simulink model "miniprojectr12"  (R2015a)
settings: Solver=ode45  StartTime=0.0  StopTime=.1  RelTol=1e-3
undefined symbols (not defined in the file): D1, Delta
libraries: powerlib x16, dspstat3 x11, powerlib_meascontrol x4
settings Model: Creator=ASUS  LastModifiedBy=ASUS

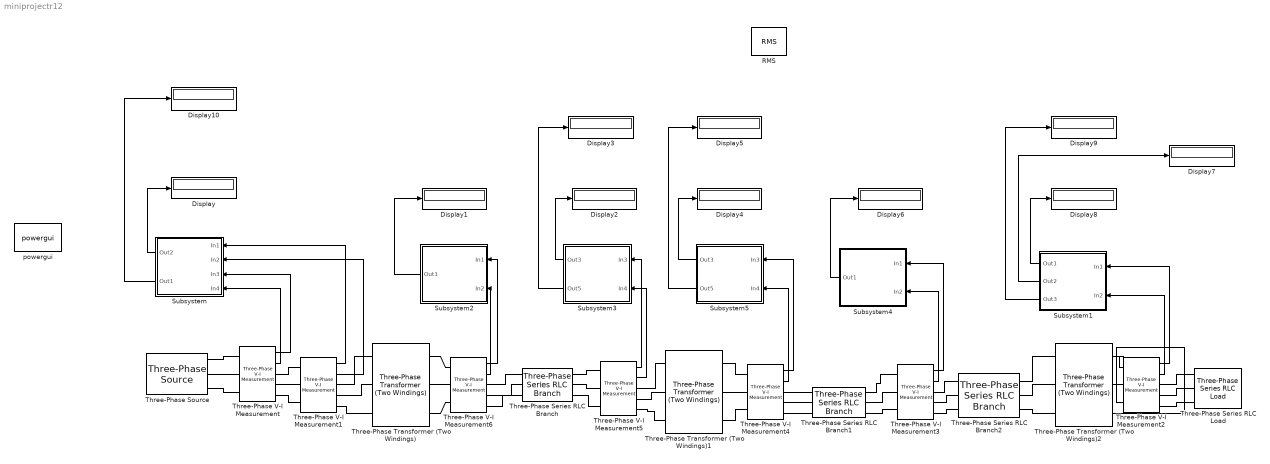
== system miniprojectr12 ==
  Display{,1..10} (11 alike) : Display
  RMS : powerlib_meascontrol/Measurements/RMS  TrueRMS=on  Freq=60  RMSInit=120  Ts=0
  Subsystem : Subsystem
  Subsystem1 : Subsystem
  Subsystem2 : Subsystem
  Subsystem3 : Subsystem
  Subsystem4 : Subsystem
  Subsystem5 : Subsystem
  Three-Phase Series RLC Branch : powerlib/Elements/Three-Phase Series RLC Branch  LConnTagsString=A|B|C  RConnTagsString=A|B|C  BranchType=RL  Resistance=271*0.01  Inductance=271*0.01  Capacitance=1e-6  Measurements=None
  Three-Phase Series RLC Branch1 : powerlib/Elements/Three-Phase Series RLC Branch  LConnTagsString=A|B|C  RConnTagsString=A|B|C  BranchType=RL  Resistance=271*0.01  Inductance=271*0.01  Capacitance=1e-6  Measurements=None
  Three-Phase Series RLC Branch2 : powerlib/Elements/Three-Phase Series RLC Branch  LConnTagsString=A|B|C  RConnTagsString=A|B|C  BranchType=RL  Resistance=271*0.01  Inductance=271*0.01  Capacitance=1e-6  Measurements=None
  Three-Phase Series RLC Load : powerlib/Elements/Three-Phase Series RLC Load  LConnTagsString=A|B|C  Configuration=Y (grounded)  NominalVoltage=1000  NominalFrequency=50  ActivePower=1e6  InductivePower=0.5e6  CapacitivePower=0  Measurements=None  LoadType=constant Z
  Three-Phase Transformer (Two Windings) : powerlib/Elements/Three-Phase Transformer (Two Windings)  Winding1Connection=Delta (D1)  Winding2Connection=Yg  CoreType=Three single-phase transformers  SetSaturation=off  Hysteresis=off  DataFile='hysteresis'  SetInitialFlux=off  Measurements=None  UNITS=pu  NominalPower=[ 250e6 , 50 ]  Winding1=[ 11e3 , 0.002 , 0.08 ]  Winding2=[ 230e3 , 0.002 , 0.08 ]  Rm=500  Lm=500  L0=0.5  Saturation=[ 0,0 ; 0.0024,1.2 ; 1.0,1.52 ]  InitialFluxes=[ 0.8 , -0.8 , 0.7 ]  MoreParameters=off  BreakLoop=off  DataType=off  TransfoNumber=1
  Three-Phase Transformer (Two Windings)1 : powerlib/Elements/Three-Phase Transformer (Two Windings)  Winding1Connection=Yg  Winding2Connection=Delta (D1)  CoreType=Three single-phase transformers  SetSaturation=off  Hysteresis=off  DataFile='hysteresis'  SetInitialFlux=off  Measurements=None  UNITS=SI  NominalPower=[ 450e6 , 50 ]  Winding1=[230e3 5.5555e-09 1.5636e-12]  Winding2=[11e3 2.7638e+09 7.7788e+05]  Rm=0.0013889  Lm=9.7726e-09  L0=2.2105e-06  Saturation=[0 0;4.3199e+08 4.2217;1.8e+11 5.3475]  InitialFluxes=[2.8144 -2.8144 2.4627]  MoreParameters=off  BreakLoop=off  DataType=on  TransfoNumber=1
  Three-Phase Transformer (Two Windings)2 : powerlib/Elements/Three-Phase Transformer (Two Windings)  Winding1Connection=Yg  Winding2Connection=Yg  CoreType=Three single-phase transformers  SetSaturation=off  Hysteresis=off  DataFile='hysteresis'  SetInitialFlux=off  Measurements=None  UNITS=pu  NominalPower=[ 450e6 , 50 ]  Winding1=[ 11000 , 0.002 , 0.08 ]  Winding2=[ 400 , 0.002 , 0.08 ]  Rm=500  Lm=500  L0=0.5  Saturation=[ 0,0 ; 0.0024,1.2 ; 1.0,1.52 ]  InitialFluxes=[ 0.8 , -0.8 , 0.7 ]  MoreParameters=off  BreakLoop=off  DataType=off  TransfoNumber=1
  Three-Phase V-I Measurement{,1..6} (7 alike) : powerlib/Measurements/Three-Phase V-I Measurement  VoltageMeasurement=phase-to-ground  SetLabelV=off  LabelV=Vabc  Vpu=off  VpuLL=off  CurrentMeasurement=yes  SetLabelI=off  LabelI=Iabc  Ipu=off  Pbase=100e6  Vbase=500e3  OutputType=Complex  PhasorSimulation=off  PSBequivalent=0
  Three-Phase Source : powerlib/Electrical Sources/Three-Phase Source  Voltage=11000  PhaseAngle=0  Frequency=50  InternalConnection=Yg  SpecifyImpedance=off  Resistance=0  Inductance=0  ShortCircuitLevel=100e6  BaseVoltage=25e3  XRratio=7  BusType=swing  Pref=0  Qref=0  Qmin=-inf  Qmax=inf
  powergui : powerlib/powergui  Priority=1  SimulationMode=Continuous  SolverType=Tustin/Backward Euler (TBE)  SampleTime=50e-6  frequency=60  SPID=off  DisableSnubberDevices=off  DisableRonSwitches=off  DisableVfSwitches=off  SwTol=0  DisplayEquations=off  Interpol=off  methode=off  Ts=100  FunctionMessages=off  echomessages=off  HookPort=off  EnableUseOfTLC=off  x0status=blocks  frequencyindice=50  Pbase=100e6  ErrMax=1e-4  Iterations=50  UnitsV=kV  UnitsW=MW  buscounter=0  RestoreLinks=warning  ResistiveCurrentMeasurement=off  Frange=[0:2:500]  Ylog=off  Xlog=on  ShowGrid=off  save=off  variable=ZData  structure=0  ZoomFFT=off  StartTime=0.0  cycles=1  DisplayStyle=1  fundamental=60  FreqAxis=off  MaxFrequency=1000  frequencyindicesteady=1  RmsSteady=1  display=off
  wires:
  Three-Phase V-I Measurement/1 -> Subsystem/3(In3)
  Three-Phase V-I Measurement/2 -> Subsystem/4(In4)
  Three-Phase V-I Measurement1/1 -> Subsystem/1(In1)
  Three-Phase V-I Measurement1/2 -> Subsystem/2(In2)
  Three-Phase V-I Measurement6/1 -> Subsystem2/1(In1)
  Three-Phase V-I Measurement6/2 -> Subsystem2/2(In2)
  Three-Phase V-I Measurement4/1 -> Subsystem5/1(In3)
  Three-Phase V-I Measurement4/2 -> Subsystem5/2(In4)
  Three-Phase V-I Measurement2/1 -> Subsystem1/1(In1)
  Three-Phase V-I Measurement2/2 -> Subsystem1/2(In2)
  Three-Phase V-I Measurement5/1 -> Subsystem3/1(In3)
  Three-Phase V-I Measurement5/2 -> Subsystem3/2(In4)
  Three-Phase V-I Measurement3/1 -> Subsystem4/1(In1)
  Three-Phase V-I Measurement3/2 -> Subsystem4/2(In2)
  Subsystem/2(Out1) -> Display10/1
  Subsystem2/1(Out1) -> Display1/1
  Subsystem3/1(Out3) -> Display2/1
  Subsystem3/2(Out5) -> Display3/1
  Subsystem5/1(Out3) -> Display4/1
  Subsystem5/2(Out5) -> Display5/1
  Subsystem4/1(Out1) -> Display6/1
  Subsystem1/1(Out1) -> Display8/1
  Subsystem1/2(Out2) -> Display7/1
  Subsystem1/3(Out3) -> Display9/1
  Subsystem/1(Out2) -> Display/1
  connections:
  Three-Phase V-I Measurement/LConn1 -- Three-Phase Source/RConn1
  Three-Phase V-I Measurement/LConn2 -- Three-Phase Source/RConn2
  Three-Phase V-I Measurement/LConn3 -- Three-Phase Source/RConn3
  Three-Phase V-I Measurement1/LConn1 -- Three-Phase V-I Measurement/RConn1
  Three-Phase V-I Measurement/RConn2 -- Three-Phase V-I Measurement1/LConn2
  Three-Phase V-I Measurement/RConn3 -- Three-Phase V-I Measurement1/LConn3
  Three-Phase Transformer (Two Windings)/LConn1 -- Three-Phase V-I Measurement1/RConn1
  Three-Phase Transformer (Two Windings)/LConn2 -- Three-Phase V-I Measurement1/RConn2
  Three-Phase Transformer (Two Windings)/LConn3 -- Three-Phase V-I Measurement1/RConn3
  Three-Phase Transformer (Two Windings)/RConn2 -- Three-Phase V-I Measurement6/LConn2
  Three-Phase Transformer (Two Windings)/RConn1 -- Three-Phase V-I Measurement6/LConn1
  Three-Phase Transformer (Two Windings)/RConn3 -- Three-Phase V-I Measurement6/LConn3
  Three-Phase Series RLC Branch/LConn1 -- Three-Phase V-I Measurement6/RConn1
  Three-Phase V-I Measurement5/LConn2 -- Three-Phase Series RLC Branch/RConn2
  Three-Phase Series RLC Branch/RConn1 -- Three-Phase V-I Measurement5/LConn1
  Three-Phase V-I Measurement5/LConn3 -- Three-Phase Series RLC Branch/RConn3
  Three-Phase V-I Measurement5/RConn1 -- Three-Phase Transformer (Two Windings)1/LConn1
  Three-Phase V-I Measurement5/RConn2 -- Three-Phase Transformer (Two Windings)1/LConn2
  Three-Phase V-I Measurement5/RConn3 -- Three-Phase Transformer (Two Windings)1/LConn3
  Three-Phase Transformer (Two Windings)1/RConn1 -- Three-Phase V-I Measurement4/LConn1
  Three-Phase Transformer (Two Windings)1/RConn2 -- Three-Phase V-I Measurement4/LConn2
  Three-Phase Transformer (Two Windings)1/RConn3 -- Three-Phase V-I Measurement4/LConn3
  Three-Phase Series RLC Branch1/LConn2 -- Three-Phase V-I Measurement4/RConn2
  Three-Phase V-I Measurement4/RConn3 -- Three-Phase Series RLC Branch1/LConn3
  Three-Phase V-I Measurement3/LConn1 -- Three-Phase Series RLC Branch1/RConn1
  Three-Phase V-I Measurement3/LConn2 -- Three-Phase Series RLC Branch1/RConn2
  Three-Phase V-I Measurement3/LConn3 -- Three-Phase Series RLC Branch1/RConn3
  Three-Phase V-I Measurement3/RConn2 -- Three-Phase Series RLC Branch2/LConn2
  Three-Phase V-I Measurement3/RConn3 -- Three-Phase Series RLC Branch2/LConn3
  Three-Phase V-I Measurement3/RConn1 -- Three-Phase Series RLC Branch2/LConn1
  Three-Phase Transformer (Two Windings)2/LConn1 -- Three-Phase Series RLC Branch2/RConn1
  Three-Phase Transformer (Two Windings)2/LConn2 -- Three-Phase Series RLC Branch2/RConn2
  Three-Phase Transformer (Two Windings)2/LConn3 -- Three-Phase Series RLC Branch2/RConn3
  Three-Phase Transformer (Two Windings)2/RConn1 -- Three-Phase V-I Measurement2/LConn1
  Three-Phase Transformer (Two Windings)2/RConn2 -- Three-Phase V-I Measurement2/LConn2
  Three-Phase Transformer (Two Windings)2/RConn3 -- Three-Phase V-I Measurement2/LConn3
  Three-Phase Series RLC Load/LConn1 -- Three-Phase V-I Measurement2/RConn1
  Three-Phase V-I Measurement2/RConn2 -- Three-Phase Series RLC Load/LConn2
  Three-Phase V-I Measurement2/RConn3 -- Three-Phase Series RLC Load/LConn3
  Three-Phase V-I Measurement4/RConn1 -- Three-Phase Series RLC Branch1/LConn1
  Three-Phase V-I Measurement6/RConn2 -- Three-Phase Series RLC Branch/LConn2
  Three-Phase V-I Measurement6/RConn3 -- Three-Phase Series RLC Branch/LConn3

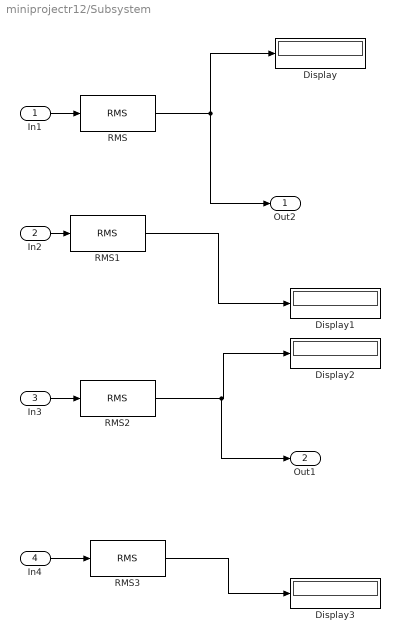
== system miniprojectr12/Subsystem ==
  In1 : Inport
  In2 : Inport  Port=2
  In3 : Inport  Port=3
  In4 : Inport  Port=4
  Display{,1..3} (4 alike) : Display
  RMS{,1..3} (4 alike) : dspstat3/RMS  run=off  reset_popup=None  InputProcessing=Columns as channels (frame based)  directionMode=Each column  dimension=1  treatSBRowAsCol=off
  Out2 : Outport
  Out1 : Outport  Port=2
  wires:
  In1/1 -> RMS/1
  RMS/1 -> Out2/1, Display/1
  In2/1 -> RMS1/1
  RMS1/1 -> Display1/1
  In3/1 -> RMS2/1
  RMS2/1 -> Out1/1, Display2/1
  In4/1 -> RMS3/1
  RMS3/1 -> Display3/1

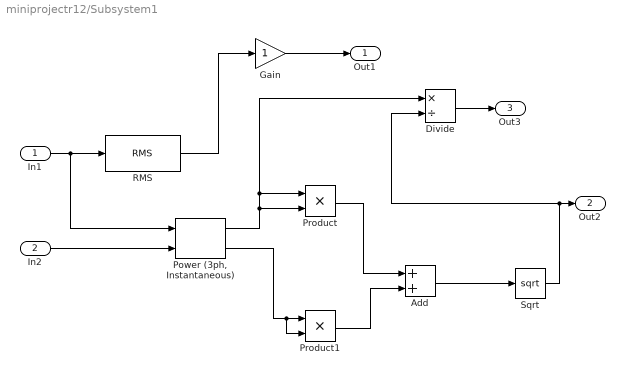
== system miniprojectr12/Subsystem1 ==
  In1 : Inport
  In2 : Inport  Port=2
  Add : Sum
  Divide : Product  Inputs=*/  SaturateOnIntegerOverflow=on  RndMeth=Zero
  Gain : Gain
  "Power (3ph, Instantaneous)" : powerlib_meascontrol/Measurements/Power (3ph, Instantaneous)
  Product : Product
  Product1 : Product
  RMS : dspstat3/RMS  run=off  reset_popup=None  InputProcessing=Columns as channels (frame based)  directionMode=Each column  dimension=1  treatSBRowAsCol=off
  Sqrt : Sqrt  SaturateOnIntegerOverflow=on
  Out1 : Outport
  Out2 : Outport  Port=2
  Out3 : Outport  Port=3
  wires:
  In1/1 -> "Power (3ph, Instantaneous)"/1, RMS/1
  Divide/1 -> Out3/1
  In2/1 -> "Power (3ph, Instantaneous)"/2
  "Power (3ph, Instantaneous)"/2 -> Product1/2, Product1/1
  Product1/1 -> Add/2
  Add/1 -> Sqrt/1
  "Power (3ph, Instantaneous)"/1 -> Divide/1, Product/1, Product/2
  Sqrt/1 -> Out2/1, Divide/2
  Gain/1 -> Out1/1
  RMS/1 -> Gain/1
  Product/1 -> Add/1

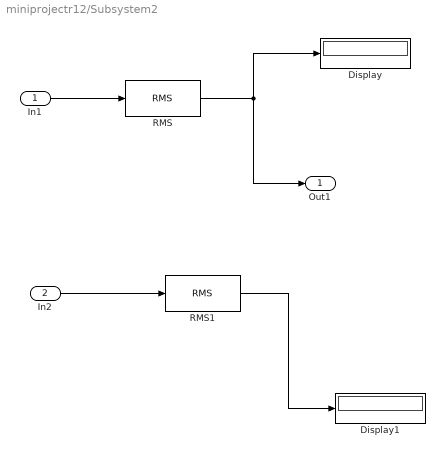
== system miniprojectr12/Subsystem2 ==
  In1 : Inport
  In2 : Inport  Port=2
  Display : Display
  Display1 : Display
  RMS : dspstat3/RMS  run=off  reset_popup=None  InputProcessing=Columns as channels (frame based)  directionMode=Each column  dimension=1  treatSBRowAsCol=off
  RMS1 : dspstat3/RMS  run=off  reset_popup=None  InputProcessing=Columns as channels (frame based)  directionMode=Each column  dimension=1  treatSBRowAsCol=off
  Out1 : Outport
  wires:
  In1/1 -> RMS/1
  RMS/1 -> Out1/1, Display/1
  In2/1 -> RMS1/1
  RMS1/1 -> Display1/1

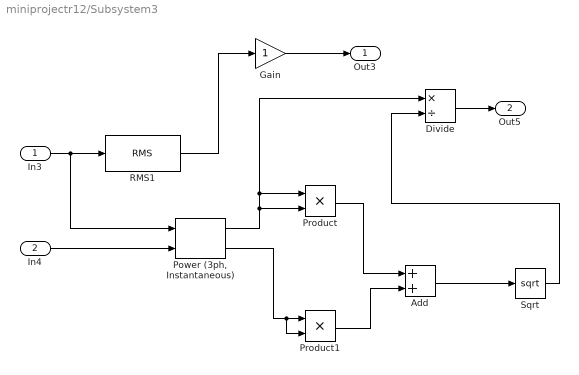
== system miniprojectr12/Subsystem3 ==
  In3 : Inport
  In4 : Inport  Port=2
  Add : Sum
  Divide : Product  Inputs=*/  SaturateOnIntegerOverflow=on  RndMeth=Zero
  Gain : Gain
  "Power (3ph, Instantaneous)" : powerlib_meascontrol/Measurements/Power (3ph, Instantaneous)
  Product : Product
  Product1 : Product
  RMS1 : dspstat3/RMS  run=off  reset_popup=None  InputProcessing=Columns as channels (frame based)  directionMode=Each column  dimension=1  treatSBRowAsCol=off
  Sqrt : Sqrt  SaturateOnIntegerOverflow=on
  Out3 : Outport
  Out5 : Outport  Port=2
  wires:
  In3/1 -> "Power (3ph, Instantaneous)"/1, RMS1/1
  Divide/1 -> Out5/1
  In4/1 -> "Power (3ph, Instantaneous)"/2
  "Power (3ph, Instantaneous)"/2 -> Product1/2, Product1/1
  Product1/1 -> Add/2
  Add/1 -> Sqrt/1
  "Power (3ph, Instantaneous)"/1 -> Divide/1, Product/1, Product/2
  Sqrt/1 -> Divide/2
  Gain/1 -> Out3/1
  RMS1/1 -> Gain/1
  Product/1 -> Add/1

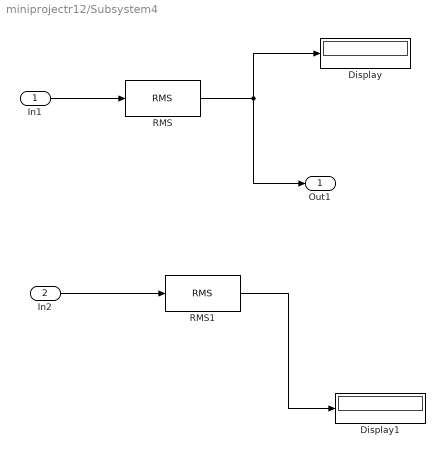
== system miniprojectr12/Subsystem4 ==
  In1 : Inport
  In2 : Inport  Port=2
  Display : Display
  Display1 : Display
  RMS : dspstat3/RMS  run=off  reset_popup=None  InputProcessing=Columns as channels (frame based)  directionMode=Each column  dimension=1  treatSBRowAsCol=off
  RMS1 : dspstat3/RMS  run=off  reset_popup=None  InputProcessing=Columns as channels (frame based)  directionMode=Each column  dimension=1  treatSBRowAsCol=off
  Out1 : Outport
  wires:
  In1/1 -> RMS/1
  RMS/1 -> Out1/1, Display/1
  In2/1 -> RMS1/1
  RMS1/1 -> Display1/1

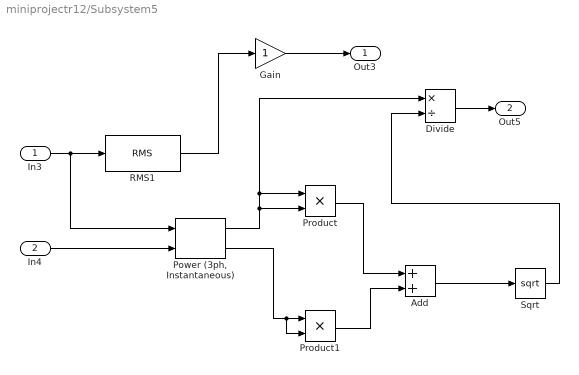
== system miniprojectr12/Subsystem5 ==
  In3 : Inport
  In4 : Inport  Port=2
  Add : Sum
  Divide : Product  Inputs=*/  SaturateOnIntegerOverflow=on  RndMeth=Zero
  Gain : Gain
  "Power (3ph, Instantaneous)" : powerlib_meascontrol/Measurements/Power (3ph, Instantaneous)
  Product : Product
  Product1 : Product
  RMS1 : dspstat3/RMS  run=off  reset_popup=None  InputProcessing=Columns as channels (frame based)  directionMode=Each column  dimension=1  treatSBRowAsCol=off
  Sqrt : Sqrt  SaturateOnIntegerOverflow=on
  Out3 : Outport
  Out5 : Outport  Port=2
  wires:
  In3/1 -> "Power (3ph, Instantaneous)"/1, RMS1/1
  Divide/1 -> Out5/1
  In4/1 -> "Power (3ph, Instantaneous)"/2
  "Power (3ph, Instantaneous)"/2 -> Product1/2, Product1/1
  Product1/1 -> Add/2
  Add/1 -> Sqrt/1
  "Power (3ph, Instantaneous)"/1 -> Divide/1, Product/1, Product/2
  Sqrt/1 -> Divide/2
  Gain/1 -> Out3/1
  RMS1/1 -> Gain/1
  Product/1 -> Add/1
